simulink model "CCCS_lin_in_diff_out_comm"  (Simulink 7.5)
settings: Solver=ode45  StartTime=0.0  StopTime=10.0  RelTol=1e-3
settings Model: Creator=tugui_cat  LastModifiedBy=tugui
settings DebuggingCC: StrictBusMsg=Warning

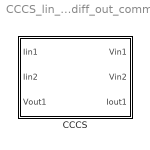
== system CCCS_lin_in_diff_out_comm ==
  CCCS : Subsystem  mask{Num_TF_dir1=1, Den_TF_dir1=1, Num_Zin1=1, Den_Zin1=1, Num_TF_inv1=1, Den_TF_inv1=1, Num_Zout1=1, Den_Zout1=1, Num_TF_dir3=1, Den_TF_dir3=1, Num_TF_inv3=1, Den_TF_inv3=1, Num_Zin_diff1=1, Den_Zin_diff1=1, Num_Zin_diff2=1, Den_Zin_diff2=1, Num_Zin2=1, Den_Zin2=1, OffIn11=0, OffIn12=0, OffIn21=0, OffIn22=0, OffOut11=0, OffOut12=0}

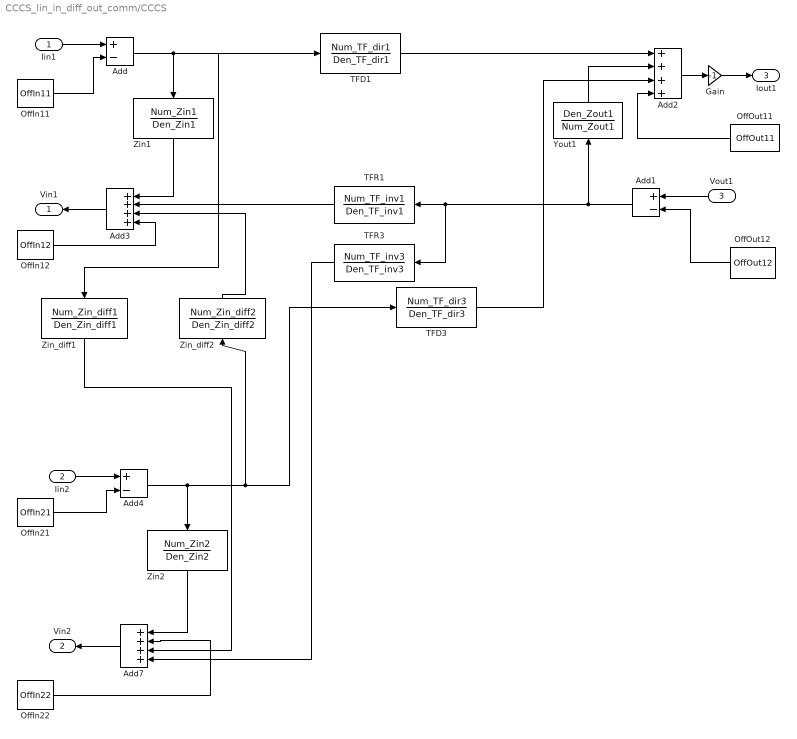
== system CCCS_lin_in_diff_out_comm/CCCS ==
  Iin1 : Inport
  Iin2 : Inport  Port=2
  Vout1 : Inport  Port=3
  Add : Sum  Inputs=+-  OutDataType=fixdt(1, 16)  OutScaling=2^-10
  Add1 : Sum  Inputs=+-  OutDataType=fixdt(1, 16)  OutScaling=2^-10
  Add2 : Sum  Inputs=++++  OutDataType=fixdt(1, 16)  OutScaling=2^-10
  Add3 : Sum  Inputs=++++  OutDataType=fixdt(1, 16)  OutScaling=2^-10
  Add4 : Sum  Inputs=+-  OutDataType=fixdt(1, 16)  OutScaling=2^-10
  Add7 : Sum  Inputs=++++  OutDataType=fixdt(1, 16)  OutScaling=2^-10
  Gain : Gain  Gain=-1  ParameterDataType=fixdt(1, 16)  ParameterScaling=2^0  OutDataType=fixdt(1, 16)  OutScaling=2^0
  OffIn11 : Constant  Value=OffIn11  OutDataType=fixdt(1, 16)  OutScaling=2^0
  OffIn12 : Constant  Value=OffIn12  OutDataType=fixdt(1, 16)  OutScaling=2^0
  OffIn21 : Constant  Value=OffIn21  OutDataType=fixdt(1, 16)  OutScaling=2^0
  OffIn22 : Constant  Value=OffIn22  OutDataType=fixdt(1, 16)  OutScaling=2^0
  OffOut11 : Constant  Value=OffOut11  OutDataType=fixdt(1, 16)  OutScaling=2^0
  OffOut12 : Constant  Value=OffOut12  OutDataType=fixdt(1, 16)  OutScaling=2^0
  TFD1 : TransferFcn  Numerator=Num_TF_dir1  Denominator=Den_TF_dir1
  TFD3 : TransferFcn  Numerator=Num_TF_dir3  Denominator=Den_TF_dir3
  TFR1 : TransferFcn  Numerator=Num_TF_inv1  Denominator=Den_TF_inv1
  TFR3 : TransferFcn  Numerator=Num_TF_inv3  Denominator=Den_TF_inv3
  Yout1 : TransferFcn  Numerator=Den_Zout1  Denominator=Num_Zout1
  Zin1 : TransferFcn  Numerator=Num_Zin1  Denominator=Den_Zin1
  Zin2 : TransferFcn  Numerator=Num_Zin2  Denominator=Den_Zin2
  Zin_diff1 : TransferFcn  Numerator=Num_Zin_diff1  Denominator=Den_Zin_diff1
  Zin_diff2 : TransferFcn  Numerator=Num_Zin_diff2  Denominator=Den_Zin_diff2
  Vin1 : Outport
  Vin2 : Outport  Port=2
  Iout1 : Outport  Port=3
  wires:
  TFD1/1 -> Add2/1
  Add3/1 -> Vin1/1
  Zin1/1 -> Add3/1
  TFR1/1 -> Add3/2
  Yout1/1 -> Add2/2
  Iin1/1 -> Add/1
  Add/1 -> Zin1/1, TFD1/1, Zin_diff1/1
  OffIn11/1 -> Add/2
  Vout1/1 -> Add1/1
  Add1/1 -> Yout1/1, TFR1/1, TFR3/1
  OffOut12/1 -> Add1/2
  Add7/1 -> Vin2/1
  Zin2/1 -> Add7/1
  Iin2/1 -> Add4/1
  Add4/1 -> Zin2/1, TFD3/1, Zin_diff2/1
  OffIn21/1 -> Add4/2
  TFD3/1 -> Add2/3
  Zin_diff1/1 -> Add7/3
  Zin_diff2/1 -> Add3/3
  OffIn12/1 -> Add3/4
  OffIn22/1 -> Add7/2
  OffOut11/1 -> Add2/4
  Add2/1 -> Gain/1
  TFR3/1 -> Add7/4
  Gain/1 -> Iout1/1
